simulink model "TestSingle"  (R2018a)
settings: Solver=FixedStepAuto  StartTime=0.0  StopTime=10  FixedStep=0.2  RelTol=1e-3  EnableMultiTasking=on
settings Model: SimulationMode=accelerator  EnablePacing=on  Creator=Hungs  LastModifiedBy=Hungs

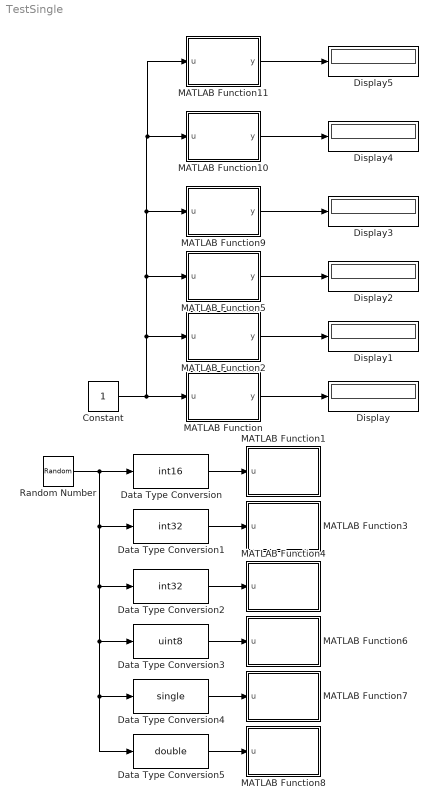
== system TestSingle ==
  Constant : Constant
  Data Type Conversion : DataTypeConversion  OutDataTypeStr=int16
  Data Type Conversion1 : DataTypeConversion  OutDataTypeStr=int32
  Data Type Conversion2 : DataTypeConversion  OutDataTypeStr=int32
  Data Type Conversion3 : DataTypeConversion  OutDataTypeStr=uint8
  Data Type Conversion4 : DataTypeConversion  OutDataTypeStr=single
  Data Type Conversion5 : DataTypeConversion  OutDataTypeStr=double
  Display{,1..5} (6 alike) : Display
      settings: Decimation=2
  MATLAB Function : MATLAB Function  TreatAsAtomicUnit=on
  MATLAB Function1 : MATLAB Function  TreatAsAtomicUnit=on
  MATLAB Function10 : MATLAB Function  TreatAsAtomicUnit=on
  MATLAB Function11 : MATLAB Function  TreatAsAtomicUnit=on
  MATLAB Function2 : MATLAB Function  TreatAsAtomicUnit=on
  MATLAB Function3 : MATLAB Function  TreatAsAtomicUnit=on
  MATLAB Function4 : MATLAB Function  TreatAsAtomicUnit=on
  MATLAB Function5 : MATLAB Function  TreatAsAtomicUnit=on
  MATLAB Function6 : MATLAB Function  TreatAsAtomicUnit=on
  MATLAB Function7 : MATLAB Function  TreatAsAtomicUnit=on
  MATLAB Function8 : MATLAB Function  TreatAsAtomicUnit=on
  MATLAB Function9 : MATLAB Function  TreatAsAtomicUnit=on
  Random Number : RandomNumber  Mean=5  Variance=5
  wires:
  MATLAB Function/1(y) -> Display/1
  MATLAB Function2/1(y) -> Display1/1
  Data Type Conversion/1 -> MATLAB Function1/1(u)
  Data Type Conversion1/1 -> MATLAB Function3/1(u)
  Data Type Conversion2/1 -> MATLAB Function4/1(u)
  MATLAB Function5/1(y) -> Display2/1
  Data Type Conversion3/1 -> MATLAB Function6/1(u)
  Data Type Conversion4/1 -> MATLAB Function7/1(u)
  Data Type Conversion5/1 -> MATLAB Function8/1(u)
  Random Number/1 -> Data Type Conversion5/1, Data Type Conversion4/1, Data Type Conversion3/1, Data Type Conversion2/1, Data Type Conversion1/1, Data Type Conversion/1
  MATLAB Function9/1(y) -> Display3/1
  MATLAB Function10/1(y) -> Display4/1
  Constant/1 -> MATLAB Function11/1(u), MATLAB Function10/1(u), MATLAB Function9/1(u), MATLAB Function5/1(u), MATLAB Function2/1(u), MATLAB Function/1(u)
  MATLAB Function11/1(y) -> Display5/1

== matlab function TestSingle/MATLAB Function ==
  data: u input; y output
function y = fcn(u)
coder.extrinsic('AdsRead');
y = int16(0);
if u==1
    y = AdsRead('', 851, 'MAIN.Value1', 'int');
end
end

== matlab function TestSingle/MATLAB Function1 ==
  data: u input
function fcn(u)
coder.extrinsic('AdsWrite');
    AdsWrite('', 851, 'MAIN.Value1', 'int', u);
end

== matlab function TestSingle/MATLAB Function2 ==
  data: u input; y output
function y = fcn(u)
coder.extrinsic('AdsRead');
y = int32(0);
if u==1
    y = AdsRead('', 851, 'MAIN.Value2', 'dint');
end
end

== matlab function TestSingle/MATLAB Function3 ==
  data: u input
function fcn(u)
coder.extrinsic('AdsWrite');
    AdsWrite('', 851, 'MAIN.Value2', 'dint', u);
end

== matlab function TestSingle/MATLAB Function4 ==
  data: u input
function fcn(u)
coder.extrinsic('AdsWrite');
    AdsWrite('', 851, 'MAIN.Value3', 'lint', u);
end

== matlab function TestSingle/MATLAB Function5 ==
  data: u input; y output
function y = fcn(u)
coder.extrinsic('AdsRead');
y = int32(0);
if u==1
    y = int32(AdsRead('', 851, 'MAIN.Value3', 'lint'));
end
end

== matlab function TestSingle/MATLAB Function6 ==
  data: u input
function fcn(u)
coder.extrinsic('AdsWrite');
    AdsWrite('', 851, 'MAIN.Value4', 'byte', u);
end

== matlab function TestSingle/MATLAB Function7 ==
  data: u input
function fcn(u)
coder.extrinsic('AdsWrite');
    AdsWrite('', 851, 'MAIN.Value5', 'real', u);
end

== matlab function TestSingle/MATLAB Function8 ==
  data: u input
function fcn(u)
coder.extrinsic('AdsWrite');
    AdsWrite('', 851, 'MAIN.Value6', 'lreal', u);
end

== matlab function TestSingle/MATLAB Function9 ==
  data: u input; y output
function y = fcn(u)
coder.extrinsic('AdsRead');
y = uint8(0);
if u==1
    y = uint8(AdsRead('', 851, 'MAIN.Value4', 'byte'));
end
end

== matlab function TestSingle/MATLAB Function10 ==
  data: u input; y output
function y = fcn(u)
coder.extrinsic('AdsRead');
y = single(0);
if u==1
    y = single(AdsRead('', 851, 'MAIN.Value5', 'real'));
end
end

== matlab function TestSingle/MATLAB Function11 ==
  data: u input; y output
function y = fcn(u)
coder.extrinsic('AdsRead');
y = double(0);
if u==1
    y = double(AdsRead('', 851, 'MAIN.Value6', 'lreal'));
end
end
